simulink model "lt2ASK"  (R2016b)
settings: Solver=VariableStepAuto  StartTime=0.0  StopTime=0.02  RelTol=1e-3
libraries: dsparch4 x2, commchan3 x1, commrandsrc3 x1
settings Model: Creator=white  LastModifiedBy=white

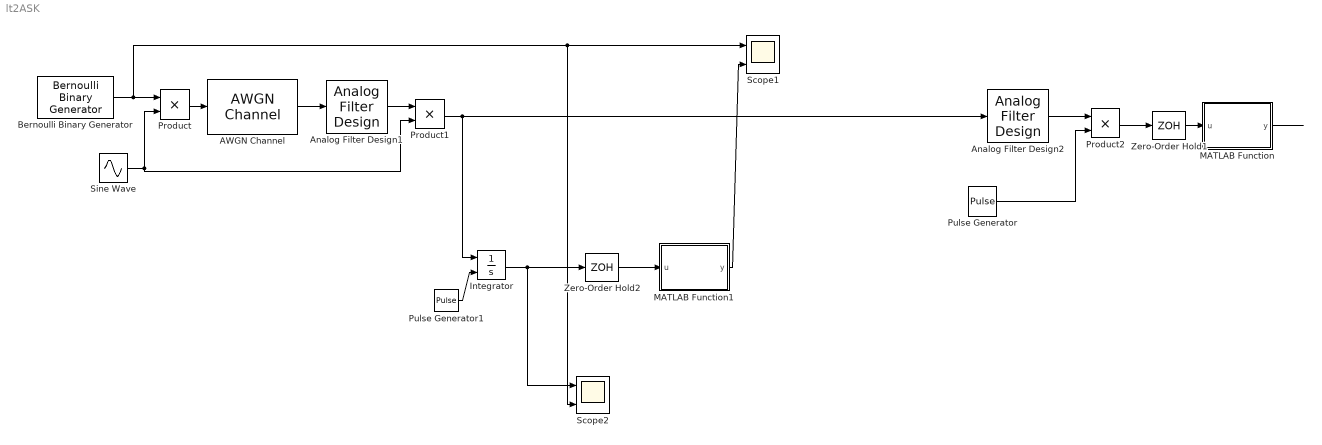
== system lt2ASK ==
  AWGN Channel : commchan3/AWGN Channel  InputProcessing=Columns as channels (frame based)  seed=67  noiseMode=Variance from mask  EbNodB=10  EsNodB=10  SNRdB=10  bitsPerSym=800  Ps=1  Tsym=1  variance=0.01
  Analog Filter Design1 : dsparch4/Analog Filter Design  method=Butterworth  filttype=Bandpass  N=1  Wlo=2*23500*pi  Whi=2*24500*pi  Rp=2  Rs=40
  Analog Filter Design2 : dsparch4/Analog Filter Design  method=Butterworth  filttype=Lowpass  N=1  Wlo=800*2*pi  Whi=2*20500*pi  Rp=2  Rs=40
  Bernoulli Binary Generator : commrandsrc3/Bernoulli Binary Generator  ProbabilityOfZero=0.5  SeedSource=Auto  Seed=0  SampleTime=0.00125  SamplesPerFrame=1  OutputDataType=double  SimulateUsing=Interpreted execution
  Integrator : Integrator  ExternalReset=rising
  MATLAB Function : MATLAB Function  TreatAsAtomicUnit=on
  MATLAB Function1 : MATLAB Function  TreatAsAtomicUnit=on
  Product : Product
  Product1 : Product
  Product2 : Product
  Pulse Generator : DiscretePulseGenerator  PulseType=Time based  Period=1/800  PulseWidth=5
  Pulse Generator1 : DiscretePulseGenerator  PulseType=Time based  Period=1/800  PulseWidth=5  PhaseDelay=1/20000
  Scope1 : Scope  NumInputPorts=2
  Scope2 : Scope  NumInputPorts=2
  Sine Wave : Sin  Frequency=24000*2*pi  SampleTime=0
  Zero-Order Hold1 : ZeroOrderHold  SampleTime=1/800
  Zero-Order Hold2 : ZeroOrderHold  SampleTime=1/800
  wires:
  Bernoulli Binary Generator/1 -> Scope2/2, Scope1/1, Product/1
  Sine Wave/1 -> Product1/2, Product/2
  Product/1 -> AWGN Channel/1
  AWGN Channel/1 -> Analog Filter Design1/1
  Analog Filter Design1/1 -> Product1/1
  Product1/1 -> Integrator/1, Analog Filter Design2/1
  Analog Filter Design2/1 -> Product2/1
  Pulse Generator/1 -> Product2/2
  Product2/1 -> Zero-Order Hold1/1
  MATLAB Function/1(y) -> ?
  Pulse Generator1/1 -> Integrator/2
  Integrator/1 -> Zero-Order Hold2/1, Scope2/1
  Zero-Order Hold2/1 -> MATLAB Function1/1(u)
  MATLAB Function1/1(y) -> Scope1/2
  Zero-Order Hold1/1 -> MATLAB Function/1(u)

== matlab function lt2ASK/MATLAB Function1 ==
  data: u input; y output
function y = fcn(u)
if(u>0.0002)
    u=1
else
    u=0
end
y = u;

== matlab function lt2ASK/MATLAB Function ==
  data: u input; y output
function y = fcn(u)
if(u>0.25)
    u=1
else
    u=0
end
y = u;
